simulink model "H41_1metro"  (R2023b)
settings: Solver=FixedStepDiscrete  StartTime=0.0  StopTime=10  FixedStep=0.01  RelTol=1e-3  EnableMultiTasking=on
model workspace (MAT data in the model file):
  d = 0.166
settings Model: ExtModeTrigDuration=2  Creator=adria  LastModifiedBy=adria
settings OptimizationCC: EnhancedBackFolding=on  PassReuseOutputArgsAs=Individual arguments  ZeroExternalMemoryAtStartup=off  ZeroInternalMemoryAtStartup=off  MaxStackSize=64  OptimizeBlockOrder=speed  DifferentSizesBufferReuse=on  EfficientTunableParamExpr=on
settings DebuggingCC: ParameterTunabilityLossMsg=error
settings HardwareCC: ProdBitPerInt=16  ProdBitPerPointer=16  ProdBitPerSizeT=16  ProdBitPerPtrDiffT=16  ProdLargestAtomicFloat=None  ProdWordSize=8  ProdHWDeviceType=Atmel->AVR  UseEmbeddedCoderFeatures=off  UseSimulinkCoderFeatures=off
settings SFSimCC: MATLABDynamicMemAlloc=off
settings RTWCC: Description=Embedded Coder  SystemTargetFile=ert.tlc  HardwareBoard=Arduino Mega 2560  TemplateMakefile=ert_default_tmf  Toolchain=Arduino AVR  BuildConfiguration=Faster Runs
settings CodeAppCC: ForceParamTrailComments=on  IgnoreCustomStorageClasses=off  OperatorAnnotations=on  SimulinkDataObjDesc=on  SFDataObjDesc=on  InsertBlockDesc=on
settings ERTTargetCC: SupportContinuousTime=on  SupportNonInlinedSFcns=on  SupportVariableSizeSignals=on  ExtModeTransport=3  ExtModeStaticAlloc=on  ExtModeAutomaticAllocSize=off  ExtModeStaticAllocSize=2048  ExtModeMexFile=ext_xcp  ExtModeIntrfLevel=Level2 - Open

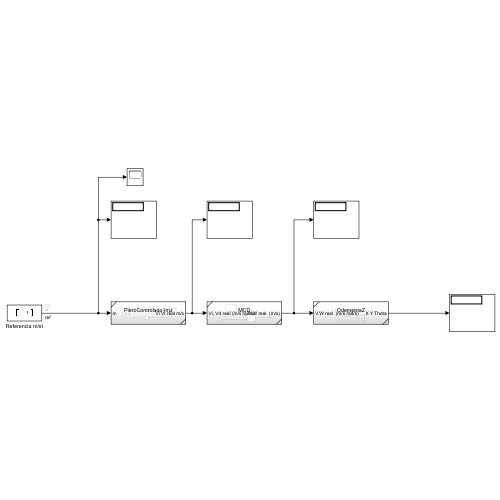
[thumbnail: Simulink's stored preview of the top-level diagram]
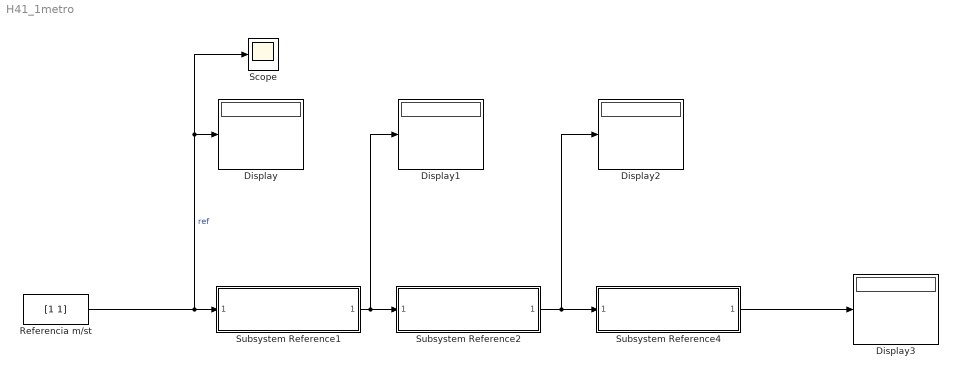
== system H41_1metro ==
  Display{,1..3} (4 alike) : Display
  Referencia m/st : Constant  Value=[1 1]
  Scope : Scope
  Subsystem Reference1 : Subsystem  ReferencedSubsystem=PieroControlado1mz
  Subsystem Reference2 : Subsystem  ReferencedSubsystem=MCD
  Subsystem Reference4 : Subsystem  ReferencedSubsystem=OdemetriaZ
  wires:
  Referencia m/st/1 -> Scope/1, Display/1, Subsystem Reference1/1  "ref"
  Subsystem Reference1/1 -> Display1/1, Subsystem Reference2/1
  Subsystem Reference2/1 -> Subsystem Reference4/1, Display2/1
  Subsystem Reference4/1 -> Display3/1
